simulink model "band_2"  (Simulink 7.8)
settings: Solver=ode45  StartTime=0.0  StopTime=10.0  RelTol=1e-3
libraries: dsparch4 x4, dspsrcs4 x1
settings Model: Creator=svenhoffmann  LastModifiedBy=josef  ExtModeAutoUpdateStatusClock=off
settings DataIOCC: SignalLoggingName=sigsOut
settings OptimizationCC: InitFltsAndDblsToZero=on
settings DebuggingCC: SaveWithParameterizedLinksMsg=none  SignalResolutionControl=TryResolveAllWithWarning  SolverPrmCheckMsg=none  MultiTaskDSMMsg=warning  MultiTaskCondExecSysMsg=none  FcnCallInpInsideContextMsg=Use local settings  StrictBusMsg=None
settings HardwareCC: TargetUnknown=on
settings RTWCC: IncludeERTFirstTime=on
settings GRTTargetCC: TargetFcnLib=ansi_tfl_tmw.mat

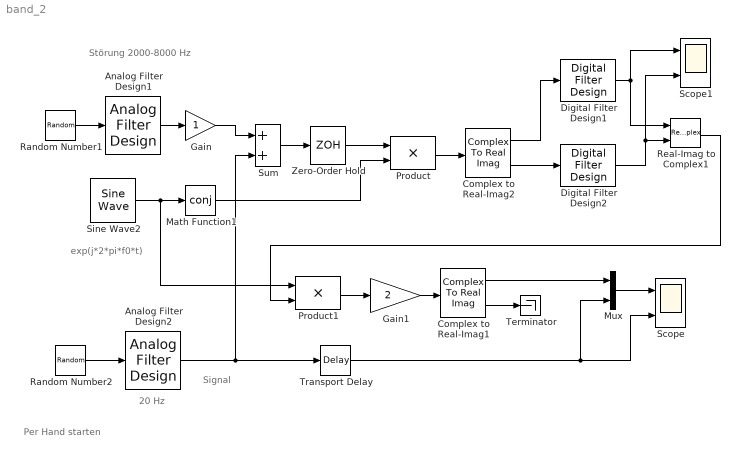
== system band_2 ==
  note: Signal
  note: exp(j*2*pi*f0*t)
  note: Störung
      | 2000-8000 Hz
  note: 20 Hz
  note: Per Hand starten
  Analog Filter Design1 : dsparch4/Analog Filter Design  method=Chebyshev I  filttype=Bandpass  N=8  Wlo=2*pi*2000  Whi=2*pi*8000  Rp=2  Rs=40
  Analog Filter Design2 : dsparch4/Analog Filter Design  method=Chebyshev I  filttype=Bandpass  N=8  Wlo=2*pi*980  Whi=2*pi*1020  Rp=2  Rs=40
  Complex to Real-Imag1 : ComplexToRealImag
  Complex to Real-Imag2 : ComplexToRealImag
  Digital Filter Design1 : dsparch4/Digital Filter Design  mwdsp_browser_bugfix_var=off
  Digital Filter Design2 : dsparch4/Digital Filter Design  mwdsp_browser_bugfix_var=off
  Gain : Gain  SaturateOnIntegerOverflow=on  OutDataTypeStr=Inherit: Same as input  ParamDataTypeStr=Inherit: Same as input
  Gain1 : Gain  Gain=2  SaturateOnIntegerOverflow=on  OutDataTypeStr=Inherit: Same as input  ParamDataTypeStr=Inherit: Same as input
  Math Function1 : Math  Operator=conj  SaturateOnIntegerOverflow=on
  Mux : Mux  Inputs=2
  Product : Product  SaturateOnIntegerOverflow=on  OutDataTypeStr=Inherit: Same as first input
  Product1 : Product  SaturateOnIntegerOverflow=on  OutDataTypeStr=Inherit: Same as first input
  Random Number1 : RandomNumber  SampleTime=0
  Random Number2 : RandomNumber  SampleTime=0
  Real-Imag to Complex1 : RealImagToComplex
  Scope : Scope  NumInputPorts=2
      settings: YMin=-0.15~-0.15  YMax=0.15~0.15  MaxDataPoints=500000
  Scope1 : Scope  NumInputPorts=2
      settings: YMin=-0.05~-0.05  YMax=0.05~0.04  MaxDataPoints=500000
  Sine Wave2 : dspsrcs4/Sine Wave  Amplitude=1  Frequency=1000  Phase=0  SampleMode=Discrete  OutComplex=Complex  CompMethod=Table lookup  TableSize=Speed  SampleTime=1/20000  SamplesPerFrame=1  ResetState=Restart at time zero  dataType=double  wordLen=16  udDataType=sfix(16)  fracBitsMode=Best precision  numFracBits=15  OutDataTypeStr=double  LastOutDataTypeStr=double
      settings: additionalParams=on
  Sum : Sum  SaturateOnIntegerOverflow=on
  Terminator : Terminator
  Transport Delay : TransportDelay  DelayTime=0.0031  BufferSize=2048
  Zero-Order Hold : ZeroOrderHold  SampleTime=1/20000
  wires:
  Analog Filter Design2/1 -> Sum/2, Transport Delay/1
  Random Number1/1 -> Analog Filter Design1/1
  Analog Filter Design1/1 -> Gain/1
  Gain/1 -> Sum/1
  Sum/1 -> Zero-Order Hold/1
  Zero-Order Hold/1 -> Product/1
  Sine Wave2/1 -> Math Function1/1, Product1/1
  Mux/1 -> Scope/1
  Transport Delay/1 -> Mux/2, Scope/2
  Product1/1 -> Gain1/1
  Gain1/1 -> Complex to Real-Imag1/1
  Product/1 -> Complex to Real-Imag2/1
  Complex to Real-Imag2/1 -> Digital Filter Design1/1
  Complex to Real-Imag2/2 -> Digital Filter Design2/1
  Digital Filter Design1/1 -> Real-Imag to Complex1/1, Scope1/1
  Digital Filter Design2/1 -> Real-Imag to Complex1/2, Scope1/2
  Real-Imag to Complex1/1 -> Product1/2
  Math Function1/1 -> Product/2
  Complex to Real-Imag1/1 -> Mux/1
  Random Number2/1 -> Analog Filter Design2/1
  Complex to Real-Imag1/2 -> Terminator/1
